simulink model "untitled"  (R2013a)
settings: Solver=ode3  StartTime=0.0  StopTime=0.01  FixedStep=0.000001  RelTol=1e-3
settings Model: Creator=Huy Hung  LastModifiedBy=Huy Hung
settings DataIOCC: InspectSignalLogs=on

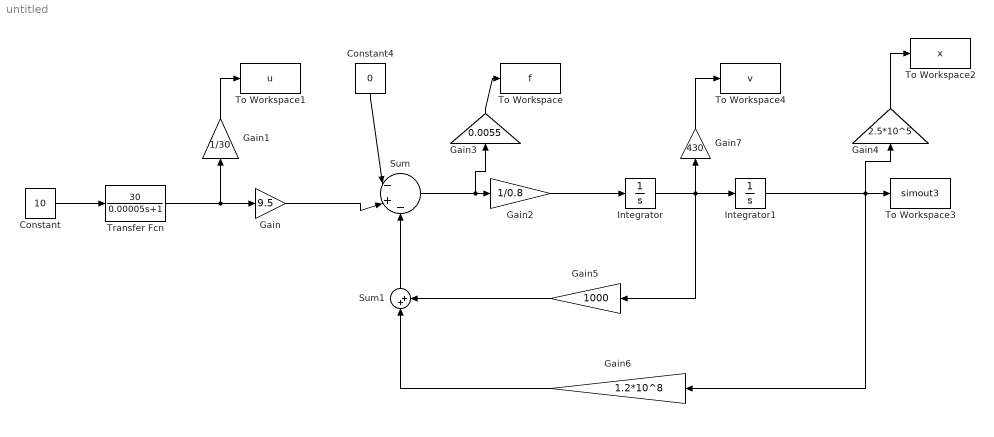
== system untitled ==
  Constant : Constant  Value=10
  Constant4 : Constant  Value=0
  Gain : Gain  Gain=9.5
  Gain1 : Gain  Gain=1/30
  Gain2 : Gain  Gain=1/0.8
  Gain3 : Gain  Gain=0.0055
  Gain4 : Gain  Gain=2.5*10^5
  Gain5 : Gain  Gain=1000
  Gain6 : Gain  Gain=1.2*10^8
  Gain7 : Gain  Gain=430
  Integrator : Integrator
  Integrator1 : Integrator
  Sum : Sum  Inputs=|-+-
  Sum1 : Sum  Inputs=|++
  To Workspace : ToWorkspace  VariableName=f  SampleTime=-1  SaveFormat=Timeseries
  To Workspace1 : ToWorkspace  VariableName=u  SampleTime=-1  SaveFormat=Timeseries
  To Workspace2 : ToWorkspace  VariableName=x  SampleTime=-1  SaveFormat=Timeseries
  To Workspace3 : ToWorkspace  VariableName=simout3  SampleTime=-1  SaveFormat=Timeseries
  To Workspace4 : ToWorkspace  VariableName=v  SampleTime=-1  SaveFormat=Timeseries
  Transfer Fcn : TransferFcn  Numerator=[30]  Denominator=[0.00005 1]
  wires:
  Constant/1 -> Transfer Fcn/1
  Transfer Fcn/1 -> Gain1/1, Gain/1
  Gain/1 -> Sum/2
  Gain1/1 -> To Workspace1/1
  Constant4/1 -> Sum/1
  Sum/1 -> Gain3/1, Gain2/1
  Gain2/1 -> Integrator/1
  Integrator/1 -> Gain7/1, Gain5/1, Integrator1/1
  Integrator1/1 -> Gain6/1, Gain4/1, To Workspace3/1
  Gain4/1 -> To Workspace2/1
  Gain3/1 -> To Workspace/1
  Gain7/1 -> To Workspace4/1
  Sum1/1 -> Sum/3
  Gain5/1 -> Sum1/2
  Gain6/1 -> Sum1/1
